simulink model "Final_EWASP_VC"  (R2022a)
settings: Solver=ode1  StartTime=0.0  StopTime=24*3600  FixedStep=10  RelTol=1e-3
values from neighbouring files (symbols this model uses):
  Aux_Threshold = 52    [Setup_Code_EWASP_VC.m]
  buildingAge = 2005    [Setup_Code_EWASP_VC.m]
  ceilingHeight = 2.4    [Setup_Code_EWASP_VC.m]
  conductiveHconnectMatrix = [ ... (first row only)    [Setup_Code_EWASP_VC.m]
  cRoofGreen = 100000    [Setup_Code_EWASP_VC.m]
  Defrost_After_Time = 30    [Setup_Code_EWASP_VC.m]
  DHWDemandProfile = occFreegainHotwaterElecTestPassiveOcc3(:,3)    [Setup_Code_EWASP_VC.m]
  Elec_Max = Elec_Max*(30/24.2)    [Setup_Code_EWASP_VC.m]
  Elec_Mid = Elec_Mid*(30/24.2)    [Setup_Code_EWASP_VC.m]
  Elec_Min = Elec_Min*(30/24.2)    [Setup_Code_EWASP_VC.m]
  ElecDemandProfile = occFreegainHotwaterElecTestPassiveOcc3(:,4)    [Setup_Code_EWASP_VC.m]
  ElecFixed = [Elec_Max(6,2) Elec_Max(6,4) Elec_Max(6,6) Elec_Max(6,7) ... (first row only)    [Setup_Code_EWASP_VC.m]
  floorOrCeilingArea = floorOrCeilingArea*1.15    [Setup_Code_EWASP_VC.m]
  forceCold = 0    [Setup_Code_EWASP_VC.m]
  freegain = occFreegainHotwaterElecTestPassiveOcc3(:,2)-max(occupancy)*25    [Setup_Code_EWASP_VC.m]
  furnitureModelOn = 1    [Setup_Code_EWASP_VC.m]
  Heat_Max = Heat_Max*(30/24.2)    [Setup_Code_EWASP_VC.m]
  Heat_Mid = Heat_Mid*(30/24.2)    [Setup_Code_EWASP_VC.m]
  Heat_Min = Heat_Min*(30/24.2)    [Setup_Code_EWASP_VC.m]
  HeatFixed = [Heat_Max(6,2) Heat_Max(6,4) Heat_Max(6,6) Heat_Max(6,7) ... (first row only)    [Setup_Code_EWASP_VC.m]
  HeatingOnProfile = repmat(HeatingOnProfile,365,1)    [Setup_Code_EWASP_VC.m]
  HEX_ReturnLowerLimit = 52.5    [Setup_Code_EWASP_VC.m]
  HEX_ReturnUpperLimit = 55    [Setup_Code_EWASP_VC.m]
  LeakMultiplier = 1+(2*(rand()-0.5)/10)    [Setup_Code_EWASP_VC.m]
  loopCap = 15    [Setup_Code_EWASP_VC.m]
  maxOcc = max(occupancyProfile)    [Setup_Code_EWASP_VC.m]
  NESW_wallArea = max(NESW_Lengths*ceilingHeight-NESW_Windows,0)    [Setup_Code_EWASP_VC.m]
  NESW_Windows = [ ... (first row only)    [Setup_Code_EWASP_VC.m]
  numRooms = roomCount    [Setup_Code_EWASP_VC.m]
  offsetDays = 0    [Setup_Code_EWASP_VC.m]
  pumpChoice = pumpChoices(MinIndex,1)    [Setup_Code_EWASP_VC.m]
  pumpRamp = 180    [Setup_Code_EWASP_VC.m]
  ReturnLowerLimit = 37.5    [Setup_Code_EWASP_VC.m]
  ReturnUpperLimit = 40    [Setup_Code_EWASP_VC.m]
  RoofIrradiance = Flat_NS_EW_RoofIrradiance(:,1)    [Setup_Code_EWASP_VC.m]
  roofStartTemp = ones(11,1)*20    [Setup_Code_EWASP_VC.m]
  rooftype = 0    [Setup_Code_EWASP_VC.m]
  RoomDataMatrix = [zeros(1,12);ones(1,12)*wallDensity;zeros(1,12);ones(1,12)*wallU;ones(1,12)*windowU;ones(1,12)*floorU;ones(1,12)*ceilingU;zeros(1,12);windowArea, 0;floorOrCeilingArea;zeros(1,12);floorOrCeilingArea*ceilingHeight]    [Setup_Code_EWASP_VC.m]
  roomVol = roomVol*1.15    [Setup_Code_EWASP_VC.m]
  slabStartTemp = (GroundTempTimeSeries(offsetDays*1440+1,1)+thermostatSetting)/2    [Setup_Code_EWASP_VC.m]
  SlackRequest = zeros(1440,1)    [Setup_Code_EWASP_VC.m]
  SolarThermalExists = 0    [Setup_Code_EWASP_VC.m]
  SourceFixed = HeatFixed-ElecFixed    [Setup_Code_EWASP_VC.m]
  StateSeries = StateSeriesGenerator(22,7,1)    [Setup_Code_EWASP_VC.m]
  Tank_Lower_Temp = 49.5    [Setup_Code_EWASP_VC.m]
  Tank_Upper_Temp = 52    [Setup_Code_EWASP_VC.m]
  Tank_Volume_m3 = 0.15    [Setup_Code_EWASP_VC.m]
  TankHeatHour = randi([1 5])-1    [Setup_Code_EWASP_VC.m]
  thermostatSetting = 20.0    (= 20)    [Setup_Code_EWASP_VC.m]
  upDown = [0;0;0;0;1;1;1;1;1;1;1]    [Setup_Code_EWASP_VC.m]
  variableASHP = 1    [Setup_Code_EWASP_VC.m]
  wallStartTempExt = thermostatSetting*(0.266+0.00215*outdoorStartTemp+0.018*wallU+0.00113*outdoorStartTemp*wallU+0.0068*wallU^2)    [Setup_Code_EWASP_VC.m]
undefined symbols (not defined in the file or in its folder): a, ceilingU, condUDMatrix, convUDMatrix, deltaPEXPANDED_E, deltaPEXPANDED_E2, deltaPEXPANDED_N, deltaPEXPANDED_N2, deltaPEXPANDED_S, deltaPEXPANDED_S2, deltaPEXPANDED_W, deltaPEXPANDED_W2, DesiredDHWTemp, DesiredFlowTempVsInOutDeltaTemp, DiffuseHorizontal, DiscIntNeverNeededParam, DNI, dwnAndConcrete, DWORK_A_HX, DWORK_CHK_FLU, DWORK_CP_NODE, DWORK_DH, DWORK_FLUID, DWORK_HCON, DWORK_LOSS, DWORK_MDOTDOWN, DWORK_MDOTIN, DWORK_MDOTUP, DWORK_MIX, DWORK_PRESS, DWORK_QDOTIN, DWORK_RHO_NODE, DWORK_TIN, DWORK_TS_OLD, DWORK_V_NODE, GroundTempTimeSeries, HCM, HCM2, HCM_closed, HCM_closed2, intermediateU, IsTop, massFlowMatrix, neighbourMatrix, numericalRoomUse, RadiatorMatrix, room2roomflowmatrix_E, room2roomflowmatrix_E2, room2roomflowmatrix_N, room2roomflowmatrix_N2, room2roomflowmatrix_S, room2roomflowmatrix_S2, room2roomflowmatrix_W, room2roomflowmatrix_W2, StateAirInEXPANDED_E, StateAirInEXPANDED_E2, StateAirInEXPANDED_N, StateAirInEXPANDED_N2, StateAirInEXPANDED_S, StateAirInEXPANDED_S2 ... (+23)
libraries: simulink x6, dspsigops x4, dspmtrx3 x4, carnot x3, spsEdgeDetectorLib x2, dspstat3 x2, powerlib_meascontrol x1, simulink_extras x1
(part 3 of 27)

== system Final_EWASP_VC/Subsystem_Room2 ==
  DNI2 : Constant  Value=0
  Diffuse Irradiance2 : Constant  Value=0
  Ground1 : Ground
  Incidence Angle2 : Constant  Value=60
  Integrator1 : Integrator  InitialConditionSource=external  InitialCondition=Tin1
  Kitchen : Subsystem
      mask Display:
      | port_label('input', 1, 'THB in')
      | port_label('input', 2, 'T In')
      | port_label('input', 3, 'T Out')
      | port_label('input', 4, 'T up (conv)')
      | port_label('input', 5, 'T Down (conv)')
      | port_label('input', 6, 'T Bel (cond)')
      | port_label('input', 7, 'T Abv (cond)')
      | port_label('input', 8, 'T N1')
      | port_label('input', 9, 'T N2')
      | port_label('input', 10, 'T N3')
      | port_label('input', 11, 'T N4')
      | port_label('input', 12, 'T N5')
      | port_label('input', 13, 'T Wall')
      | port_label('input', 14, 'Ang')
      | port_label('input', 15, 'Tilt')
      | port_label('input', 16, 'DNI')
      | port_label('input', 17, 'DiffI')
      | 
      | port_label('output', 1, 'THB Out')
      | 
      | port_label('output', 2, 'DeltaT Room')
      | 
      | port_label('input', 18, 'm_dot_Fully_open')
      | port_label('output', 3, 'm_dot_Actual')
  Panel TIlt2 : Constant  Value=90
  Subsystem10 : Subsystem
      mask Display:
      | disp('Vertical \n Conductive \n Signalling \n Block')
      | port_label('input', 1, 'Bel1')
      | port_label('input', 2, 'Bel2')
      | port_label('input', 3, 'Abv1')
      | port_label('input', 4, 'Abv2')
      | 
      | port_label('output', 1, 'T Bel')
      | port_label('output', 2, 'T Abv')
  Subsystem4 : Subsystem
      mask Display:
      | disp('Horizontal \n Neighbour \n Signalling \n Block')
      | port_label('input', 1, 'Nbr1')
      | port_label('input', 2, 'Nbr2')
      | port_label('input', 3, 'Nbr3')
      | port_label('input', 4, 'Nbr4')
      | port_label('input', 5, 'Nbr5')
      | port_label('output', 1, 'TN1')
      | port_label('output', 2, 'TN2')
      | port_label('output', 3, 'TN3')
      | port_label('output', 4, 'TN4')
      | port_label('output', 5, 'TN5')
  Terminator : Terminator
  Tinitial2 : Constant  Value=18
  Twall10 : Constant  Value=condUDMatrix(2,2)
  Twall128 : Constant  Value=neighbourMatrix(1,2)
  Twall129 : Constant  Value=neighbourMatrix(2,2)
  Twall130 : Constant  Value=neighbourMatrix(3,2)
  Twall131 : Constant  Value=neighbourMatrix(4,2)
  Twall132 : Constant  Value=neighbourMatrix(5,2)
  Twall31 : Constant  Value=condUDMatrix(3,3)
  Twall32 : Constant  Value=condUDMatrix(4,4)
  Twall9 : Constant  Value=condUDMatrix(1,2)
  tag scope: DeltaT_2=global, Mdot_Actual_2=global, T_2=global, T_return_R2=global
  wires:
  Subsystem10/2(Out2) -> Kitchen/7(In7)
  Twall9/1 -> Subsystem10/1(In1)
  Diffuse Irradiance2/1 -> Kitchen/17(In17)
  Twall10/1 -> Subsystem10/2(In2)
  Ground1/1 -> Kitchen/13(In13)
  [T_2] -> Kitchen/2(In2)
  [T_2] -> Kitchen/4(In4), Kitchen/5(In5)
  Subsystem4/3(Out3) -> Kitchen/10(In10)
  Subsystem10/1(Out1) -> Kitchen/6(In6)
  Twall32/1 -> Subsystem10/4(In4)
  [T_Out] -> Kitchen/3(In3)
  Incidence Angle2/1 -> Kitchen/14(In14)
  Twall31/1 -> Subsystem10/3(In3)
  Subsystem4/1(Out1) -> Kitchen/8(In8)
  Tinitial2/1 -> Integrator1/2
  Twall132/1 -> Subsystem4/5(In5)
  [DeltaT_2] -> Integrator1/1
  Twall130/1 -> Subsystem4/3(In3)
  Subsystem4/5(Out5) -> Kitchen/12(In12)
  Kitchen/2(Out3) -> [DeltaT_2]
  Kitchen/3(Out4) -> [Mdot_Actual_2]
  Kitchen/1(Out1) -> [T_return_R2]
  [MassFlow_Full_Open_2] -> Kitchen/18(In18)
  DNI2/1 -> Kitchen/16(In16)
  Subsystem4/2(Out2) -> Kitchen/9(In9)
  [THB_In] -> Kitchen/1(In1)
  Twall128/1 -> Subsystem4/1(In1)
  Twall131/1 -> Subsystem4/4(In4)
  Panel TIlt2/1 -> Kitchen/15(In15)
  Twall129/1 -> Subsystem4/2(In2)
  Integrator1/1 -> [T_2]
  Kitchen/4(Out2) -> Terminator/1
  Subsystem4/4(Out4) -> Kitchen/11(In11)

== system Final_EWASP_VC/Subsystem_Room3 ==
  DNI3 : Constant  Value=0
  Diffuse Irradiance3 : Constant  Value=50
  Ground2 : Ground
  Incidence Angle3 : Constant  Value=60
  Integrator5 : Integrator  InitialConditionSource=external  InitialCondition=Tin1
  Panel TIlt3 : Constant  Value=90
  Subsystem5 : Subsystem
      mask Display:
      | disp('Horizontal \n Neighbour \n Signalling \n Block')
      | port_label('input', 1, 'Nbr1')
      | port_label('input', 2, 'Nbr2')
      | port_label('input', 3, 'Nbr3')
      | port_label('input', 4, 'Nbr4')
      | port_label('input', 5, 'Nbr5')
      | port_label('output', 1, 'TN1')
      | port_label('output', 2, 'TN2')
      | port_label('output', 3, 'TN3')
      | port_label('output', 4, 'TN4')
      | port_label('output', 5, 'TN5')
  Subsystem9 : Subsystem
      mask Display:
      | disp('Vertical \n Conductive \n Signalling \n Block')
      | port_label('input', 1, 'Bel1')
      | port_label('input', 2, 'Bel2')
      | port_label('input', 3, 'Abv1')
      | port_label('input', 4, 'Abv2')
      | 
      | port_label('output', 1, 'T Bel')
      | port_label('output', 2, 'T Abv')
  Terminator11 : Terminator
  Tinitial3 : Constant  Value=18
  Twall16 : Constant  Value=neighbourMatrix(1,3)
  Twall17 : Constant  Value=neighbourMatrix(2,3)
  Twall18 : Constant  Value=neighbourMatrix(3,3)
  Twall19 : Constant  Value=neighbourMatrix(4,3)
  Twall20 : Constant  Value=neighbourMatrix(5,3)
  Twall5 : Constant  Value=condUDMatrix(1,3)
  Twall6 : Constant  Value=condUDMatrix(2,3)
  Twall7 : Constant  Value=condUDMatrix(3,3)
  Twall8 : Constant  Value=condUDMatrix(4,3)
  Utility : Subsystem
      mask Display:
      | port_label('input', 1, 'THB in')
      | port_label('input', 2, 'T In')
      | port_label('input', 3, 'T Out')
      | port_label('input', 4, 'T up (conv)')
      | port_label('input', 5, 'T Down (conv)')
      | port_label('input', 6, 'T Bel (cond)')
      | port_label('input', 7, 'T Abv (cond)')
      | port_label('input', 8, 'T N1')
      | port_label('input', 9, 'T N2')
      | port_label('input', 10, 'T N3')
      | port_label('input', 11, 'T N4')
      | port_label('input', 12, 'T N5')
      | port_label('input', 13, 'T Wall')
      | port_label('input', 14, 'Ang')
      | port_label('input', 15, 'Tilt')
      | port_label('input', 16, 'DNI')
      | port_label('input', 17, 'DiffI')
      | 
      | port_label('output', 1, 'THB Out')
      | port_label('output', 2, 'DeltaT Wall')
      | port_label('output', 3, 'DeltaT Room')
      | 
      | port_label('input', 18, 'm_dot_Fully_open')
      | port_label('output', 4, 'm_dot_Actual')
  tag scope: DeltaT_3=global, Mdot_Actual_3=global, T_3=global, T_return_R3=global
  wires:
  Ground2/1 -> Utility/13(In13)
  Subsystem5/3(Out3) -> Utility/10(In10)
  Twall5/1 -> Subsystem9/1(In1)
  Twall8/1 -> Subsystem9/4(In4)
  Twall6/1 -> Subsystem9/2(In2)
  Utility/2(Out2) -> Terminator11/1
  Twall7/1 -> Subsystem9/3(In3)
  [T_3] -> Utility/2(In2)
  Subsystem9/1(Out1) -> Utility/6(In6)
  Subsystem9/2(Out2) -> Utility/7(In7)
  Diffuse Irradiance3/1 -> Utility/17(In17)
  Integrator5/1 -> [T_3]
  Twall18/1 -> Subsystem5/3(In3)
  Incidence Angle3/1 -> Utility/14(In14)
  DNI3/1 -> Utility/16(In16)
  Panel TIlt3/1 -> Utility/15(In15)
  [THB_In] -> Utility/1(In1)
  Tinitial3/1 -> Integrator5/2
  Twall20/1 -> Subsystem5/5(In5)
  [T_Out] -> Utility/3(In3)
  [T_3] -> Utility/5(In5), Utility/4(In4)
  [MassFlow_Full_Open_3] -> Utility/18(In18)
  Utility/4(Out4) -> [Mdot_Actual_3]
  Utility/1(Out1) -> [T_return_R3]
  Twall16/1 -> Subsystem5/1(In1)
  Subsystem5/4(Out4) -> Utility/11(In11)
  Twall17/1 -> Subsystem5/2(In2)
  Subsystem5/2(Out2) -> Utility/9(In9)
  Utility/3(Out3) -> [DeltaT_3]
  Subsystem5/5(Out5) -> Utility/12(In12)
  [DeltaT_3] -> Integrator5/1
  Subsystem5/1(Out1) -> Utility/8(In8)
  Twall19/1 -> Subsystem5/4(In4)

== system Final_EWASP_VC/Subsystem_Room4 ==
  DNI11 : Constant  Value=0
  Diffuse Irradiance8 : Constant  Value=50
  Ground3 : Ground
  Hall : Subsystem
      mask Display:
      | port_label('input', 1, 'THB in')
      | port_label('input', 2, 'T In')
      | port_label('input', 3, 'T Out')
      | port_label('input', 4, 'T up (conv)')
      | port_label('input', 5, 'T Down (conv)')
      | port_label('input', 6, 'T Bel (cond)')
      | port_label('input', 7, 'T Abv (cond)')
      | port_label('input', 8, 'T N1')
      | port_label('input', 9, 'T N2')
      | port_label('input', 10, 'T N3')
      | port_label('input', 11, 'T N4')
      | port_label('input', 12, 'T N5')
      | port_label('input', 13, 'T Wall')
      | port_label('input', 14, 'Ang')
      | port_label('input', 15, 'Tilt')
      | port_label('input', 16, 'DNI')
      | port_label('input', 17, 'DiffI')
      | 
      | port_label('output', 1, 'THB Out')
      | port_label('output', 2, 'DeltaT Wall')
      | port_label('output', 3, 'DeltaT Room')
      | 
      | 
      | port_label('input', 18, 'm_dot_Fully_open')
      | port_label('output', 4, 'm_dot_Actual')
  Incidence Angle8 : Constant  Value=60
  Integrator21 : Integrator  InitialConditionSource=external  InitialCondition=Tin1
  Panel TIlt8 : Constant  Value=90
  Subsystem6 : Subsystem
      mask Display:
      | disp('Horizontal \n Neighbour \n Signalling \n Block')
      | port_label('input', 1, 'Nbr1')
      | port_label('input', 2, 'Nbr2')
      | port_label('input', 3, 'Nbr3')
      | port_label('input', 4, 'Nbr4')
      | port_label('input', 5, 'Nbr5')
      | port_label('output', 1, 'TN1')
      | port_label('output', 2, 'TN2')
      | port_label('output', 3, 'TN3')
      | port_label('output', 4, 'TN4')
      | port_label('output', 5, 'TN5')
  Subsystem8 : Subsystem
      mask Display:
      | disp('Vertical \n Conductive \n Signalling \n Block')
      | port_label('input', 1, 'Bel1')
      | port_label('input', 2, 'Bel2')
      | port_label('input', 3, 'Abv1')
      | port_label('input', 4, 'Abv2')
      | 
      | port_label('output', 1, 'T Bel')
      | port_label('output', 2, 'T Abv')
  Terminator10 : Terminator
  Tinitial11 : Constant  Value=18
  Twall1 : Constant  Value=condUDMatrix(1,4)
  Twall2 : Constant  Value=condUDMatrix(2,4)
  Twall21 : Constant  Value=neighbourMatrix(1,4)
  Twall22 : Constant  Value=neighbourMatrix(2,4)
  Twall23 : Constant  Value=neighbourMatrix(3,4)
  Twall24 : Constant  Value=neighbourMatrix(4,4)
  Twall25 : Constant  Value=neighbourMatrix(5,4)
  Twall3 : Constant  Value=condUDMatrix(3,4)
  Twall4 : Constant  Value=condUDMatrix(4,4)
  tag scope: DeltaT_4=global, Mdot_Actual_4=global, T_4=global, T_return_R4=global
  wires:
  Subsystem8/2(Out2) -> Hall/7(In7)
  Integrator21/1 -> [T_4]
  Subsystem6/1(Out1) -> Hall/8(In8)
  Ground3/1 -> Hall/13(In13)
  [DeltaT_4] -> Integrator21/1
  Incidence Angle8/1 -> Hall/14(In14)
  Subsystem8/1(Out1) -> Hall/6(In6)
  Panel TIlt8/1 -> Hall/15(In15)
  [THB_In] -> Hall/1(In1)
  Twall21/1 -> Subsystem6/1(In1)
  DNI11/1 -> Hall/16(In16)
  Diffuse Irradiance8/1 -> Hall/17(In17)
  Hall/4(Out4) -> [Mdot_Actual_4]
  Hall/3(Out3) -> [DeltaT_4]
  Twall25/1 -> Subsystem6/5(In5)
  [MassFlow_Full_Open_4] -> Hall/18(In18)
  Twall23/1 -> Subsystem6/3(In3)
  Subsystem6/5(Out5) -> Hall/12(In12)
  Twall4/1 -> Subsystem8/4(In4)
  Twall2/1 -> Subsystem8/2(In2)
  [T_4] -> Hall/5(In5)
  Hall/2(Out2) -> Terminator10/1
  [T_4] -> Hall/2(In2)
  Subsystem6/4(Out4) -> Hall/11(In11)
  Subsystem6/3(Out3) -> Hall/10(In10)
  Twall24/1 -> Subsystem6/4(In4)
  Twall22/1 -> Subsystem6/2(In2)
  Hall/1(Out1) -> [T_return_R4]
  Subsystem6/2(Out2) -> Hall/9(In9)
  Tinitial11/1 -> Integrator21/2
  [T_5] -> Hall/4(In4)
  Twall1/1 -> Subsystem8/1(In1)
  [T_Out] -> Hall/3(In3)
  Twall3/1 -> Subsystem8/3(In3)

== system Final_EWASP_VC/Subsystem_Room5 ==
  DNI4 : Constant  Value=0
  Diffuse Irradiance4 : Constant  Value=0
  Ground4 : Ground
  Incidence Angle4 : Constant  Value=60
  Integrator6 : Integrator  InitialConditionSource=external  InitialCondition=Tin1
  Landing : Subsystem
      mask Display:
      | port_label('input', 1, 'THB in')
      | port_label('input', 2, 'T In')
      | port_label('input', 3, 'T Out')
      | port_label('input', 4, 'T up (conv)')
      | port_label('input', 5, 'T Down (conv)')
      | port_label('input', 6, 'T Bel (cond)')
      | port_label('input', 7, 'T Abv (cond)')
      | port_label('input', 8, 'T N1')
      | port_label('input', 9, 'T N2')
      | port_label('input', 10, 'T N3')
      | port_label('input', 11, 'T N4')
      | port_label('input', 12, 'T N5')
      | port_label('input', 13, 'T Wall')
      | port_label('input', 14, 'Ang')
      | port_label('input', 15, 'Tilt')
      | port_label('input', 16, 'DNI')
      | port_label('input', 17, 'DiffI')
      | 
      | port_label('output', 1, 'THB Out')
      | port_label('output', 2, 'DeltaT Wall')
      | port_label('output', 3, 'DeltaT Room')
      | 
      | port_label('input', 18, 'm_dot_Fully_open')
      | port_label('output', 5, 'm_dot_Actual')
  Panel TIlt4 : Constant  Value=90
  Subsystem18 : Subsystem
      mask Display:
      | disp('Vertical \n Convective \n Signalling \n Block')
      | port_label('input', 1, 'Nbr1')
      | port_label('input', 2, 'Nbr2')
      | 
      | port_label('output', 1, 'Tup')
      | port_label('output', 2, 'Tdwn')
  Subsystem35 : Subsystem
      mask Display:
      | disp('Vertical \n Conductive \n Signalling \n Block')
      | port_label('input', 1, 'Bel1')
      | port_label('input', 2, 'Bel2')
      | port_label('input', 3, 'Abv1')
      | port_label('input', 4, 'Abv2')
      | 
      | port_label('output', 1, 'T Bel')
      | port_label('output', 2, 'T Abv')
  Subsystem7 : Subsystem
      mask Display:
      | disp('Horizontal \n Neighbour \n Signalling \n Block')
      | port_label('input', 1, 'Nbr1')
      | port_label('input', 2, 'Nbr2')
      | port_label('input', 3, 'Nbr3')
      | port_label('input', 4, 'Nbr4')
      | port_label('input', 5, 'Nbr5')
      | port_label('output', 1, 'TN1')
      | port_label('output', 2, 'TN2')
      | port_label('output', 3, 'TN3')
      | port_label('output', 4, 'TN4')
      | port_label('output', 5, 'TN5')
  Terminator12 : Terminator
  Terminator9 : Terminator
  Tinitial4 : Constant  Value=18
  Twall104 : Constant  Value=convUDMatrix(1,5)
  Twall105 : Constant  Value=convUDMatrix(2,5)
  Twall119 : Constant  Value=condUDMatrix(1,5)
  Twall120 : Constant  Value=condUDMatrix(2,5)
  Twall121 : Constant  Value=condUDMatrix(3,5)
  Twall122 : Constant  Value=condUDMatrix(4,5)
  Twall26 : Constant  Value=neighbourMatrix(1,5)
  Twall27 : Constant  Value=neighbourMatrix(2,5)
  Twall28 : Constant  Value=neighbourMatrix(3,5)
  Twall29 : Constant  Value=neighbourMatrix(4,5)
  Twall30 : Constant  Value=neighbourMatrix(5,5)
  tag scope: DeltaT_5=global, Mdot_Actual_5=global, T_5=global, T_return_R5=global
  wires:
  DNI4/1 -> Landing/16(In16)
  Twall120/1 -> Subsystem35/2(In2)
  Tinitial4/1 -> Integrator6/2
  [DeltaT_5] -> Integrator6/1
  Landing/3(Out3) -> [DeltaT_5]
  Subsystem7/5(Out5) -> Landing/12(In12)
  Integrator6/1 -> [T_5]
  Subsystem7/1(Out1) -> Landing/8(In8)
  Twall119/1 -> Subsystem35/1(In1)
  Diffuse Irradiance4/1 -> Landing/17(In17)
  Panel TIlt4/1 -> Landing/15(In15)
  [THB_In] -> Landing/1(In1)
  [T_Out] -> Landing/3(In3)
  Landing/5(Out5) -> [Mdot_Actual_5]
  Incidence Angle4/1 -> Landing/14(In14)
  Subsystem35/1(Out1) -> Landing/6(In6)
  Twall26/1 -> Subsystem7/1(In1)
  [T_5] -> Landing/2(In2)
  Ground4/1 -> Landing/13(In13)
  Subsystem7/3(Out3) -> Landing/10(In10)
  [MassFlow_Full_Open_5] -> Landing/18(In18)
  Twall27/1 -> Subsystem7/2(In2)
  Twall121/1 -> Subsystem35/3(In3)
  Subsystem18/2(Out2) -> Landing/5(In5)
  Subsystem18/1(Out1) -> Landing/4(In4)
  Twall122/1 -> Subsystem35/4(In4)
  Landing/4(Out4) -> Terminator12/1
  Landing/2(Out2) -> Terminator9/1
  Twall105/1 -> Subsystem18/2(In2)
  Subsystem7/4(Out4) -> Landing/11(In11)
  Subsystem35/2(Out2) -> Landing/7(In7)
  Landing/1(Out1) -> [T_return_R5]
  Twall30/1 -> Subsystem7/5(In5)
  Twall28/1 -> Subsystem7/3(In3)
  Twall104/1 -> Subsystem18/1(In1)
  Twall29/1 -> Subsystem7/4(In4)
  Subsystem7/2(Out2) -> Landing/9(In9)

== system Final_EWASP_VC/Subsystem_Room6 ==
  Bedroom1 : Subsystem
      mask Display:
      | port_label('input', 1, 'THB in')
      | port_label('input', 2, 'T In')
      | port_label('input', 3, 'T Out')
      | port_label('input', 4, 'T up (conv)')
      | port_label('input', 5, 'T Down (conv)')
      | port_label('input', 6, 'T Bel (cond)')
      | port_label('input', 7, 'T Abv (cond)')
      | port_label('input', 8, 'T N1')
      | port_label('input', 9, 'T N2')
      | port_label('input', 10, 'T N3')
      | port_label('input', 11, 'T N4')
      | port_label('input', 12, 'T N5')
      | port_label('input', 13, 'T Wall')
      | port_label('input', 14, 'Ang')
      | port_label('input', 15, 'Tilt')
      | port_label('input', 16, 'DNI')
      | port_label('input', 17, 'DiffI')
      | 
      | port_label('output', 1, 'THB Out')
      | port_label('output', 2, 'DeltaT Wall')
      | port_label('output', 3, 'DeltaT Room')
      | 
      | port_label('input', 18, 'm_dot_Fully_open')
      | port_label('output', 5, 'm_dot_Actual')
  DNI5 : Constant  Value=0
  Diffuse Irradiance5 : Constant  Value=0
  Ground10 : Ground
  Incidence Angle5 : Constant  Value=60
  Integrator7 : Integrator  InitialConditionSource=external  InitialCondition=Tin1
  Panel TIlt5 : Constant  Value=90
  Scope38 : Scope
  Subsystem19 : Subsystem
      mask Display:
      | disp('Vertical \n Convective \n Signalling \n Block')
      | port_label('input', 1, 'Nbr1')
      | port_label('input', 2, 'Nbr2')
      | 
      | port_label('output', 1, 'Tup')
      | port_label('output', 2, 'Tdwn')
  Subsystem30 : Subsystem
      mask Display:
      | disp('Vertical \n Conductive \n Signalling \n Block')
      | port_label('input', 1, 'Bel1')
      | port_label('input', 2, 'Bel2')
      | port_label('input', 3, 'Abv1')
      | port_label('input', 4, 'Abv2')
      | 
      | port_label('output', 1, 'T Bel')
      | port_label('output', 2, 'T Abv')
  Subsystem8 : Subsystem
      mask Display:
      | disp('Horizontal \n Neighbour \n Signalling \n Block')
      | port_label('input', 1, 'Nbr1')
      | port_label('input', 2, 'Nbr2')
      | port_label('input', 3, 'Nbr3')
      | port_label('input', 4, 'Nbr4')
      | port_label('input', 5, 'Nbr5')
      | port_label('output', 1, 'TN1')
      | port_label('output', 2, 'TN2')
      | port_label('output', 3, 'TN3')
      | port_label('output', 4, 'TN4')
      | port_label('output', 5, 'TN5')
  Terminator4 : Terminator
  Tinitial5 : Constant  Value=18
  Twall108 : Constant  Value=condUDMatrix(1,6)
  Twall109 : Constant  Value=condUDMatrix(2,6)
  Twall110 : Constant  Value=condUDMatrix(3,6)
  Twall111 : Constant  Value=condUDMatrix(4,6)
  Twall31 : Constant  Value=neighbourMatrix(1,6)
  Twall32 : Constant  Value=neighbourMatrix(2,6)
  Twall33 : Constant  Value=neighbourMatrix(3,6)
  Twall34 : Constant  Value=neighbourMatrix(4,6)
  Twall35 : Constant  Value=neighbourMatrix(5,6)
  Twall74 : Constant  Value=convUDMatrix(1,6)
  Twall75 : Constant  Value=convUDMatrix(2,6)
  tag scope: DeltaT_6=global, Mdot_Actual_6=global, T_6=global, T_return_R6=global
  wires:
  Twall75/1 -> Subsystem19/2(In2)
  Subsystem8/1(Out1) -> Bedroom1/8(In8)
  DNI5/1 -> Bedroom1/16(In16)
  Subsystem19/2(Out2) -> Bedroom1/5(In5)
  [THB_In] -> Bedroom1/1(In1)
  Integrator7/1 -> [T_6]
  [T_6] -> Bedroom1/2(In2)
  Twall31/1 -> Subsystem8/1(In1)
  [DeltaT_6] -> Integrator7/1
  Subsystem19/1(Out1) -> Bedroom1/4(In4)
  Twall34/1 -> Subsystem8/4(In4)
  Incidence Angle5/1 -> Bedroom1/14(In14)
  Twall108/1 -> Subsystem30/1(In1)
  Ground10/1 -> Bedroom1/13(In13)
  [T_Out] -> Bedroom1/3(In3)
  Panel TIlt5/1 -> Bedroom1/15(In15)
  Bedroom1/3(Out3) -> [DeltaT_6]
  Bedroom1/4(Out4) -> Scope38/1
  Tinitial5/1 -> Integrator7/2
  Bedroom1/5(Out5) -> [Mdot_Actual_6]
  Bedroom1/1(Out1) -> [T_return_R6]
  [MassFlow_Full_Open_6] -> Bedroom1/18(In18)
  Twall110/1 -> Subsystem30/3(In3)
  Subsystem8/3(Out3) -> Bedroom1/10(In10)
  Subsystem8/2(Out2) -> Bedroom1/9(In9)
  Subsystem8/5(Out5) -> Bedroom1/12(In12)
  Twall35/1 -> Subsystem8/5(In5)
  Twall32/1 -> Subsystem8/2(In2)
  Twall111/1 -> Subsystem30/4(In4)
  Twall74/1 -> Subsystem19/1(In1)
  Diffuse Irradiance5/1 -> Bedroom1/17(In17)
  Twall33/1 -> Subsystem8/3(In3)
  Subsystem8/4(Out4) -> Bedroom1/11(In11)
  Subsystem30/1(Out1) -> Bedroom1/6(In6)
  Bedroom1/2(Out2) -> Terminator4/1
  Twall109/1 -> Subsystem30/2(In2)
  Subsystem30/2(Out2) -> Bedroom1/7(In7)

== system Final_EWASP_VC/Subsystem_Room7 ==
  Bedroom 2 : Subsystem
      mask Display:
      | port_label('input', 1, 'THB in')
      | port_label('input', 2, 'T In')
      | port_label('input', 3, 'T Out')
      | port_label('input', 4, 'T up (conv)')
      | port_label('input', 5, 'T Down (conv)')
      | port_label('input', 6, 'T Bel (cond)')
      | port_label('input', 7, 'T Abv (cond)')
      | port_label('input', 8, 'T N1')
      | port_label('input', 9, 'T N2')
      | port_label('input', 10, 'T N3')
      | port_label('input', 11, 'T N4')
      | port_label('input', 12, 'T N5')
      | port_label('input', 13, 'T Wall')
      | port_label('input', 14, 'Ang')
      | port_label('input', 15, 'Tilt')
      | port_label('input', 16, 'DNI')
      | port_label('input', 17, 'DiffI')
      | 
      | port_label('output', 1, 'THB Out')
      | port_label('output', 2, 'DeltaT Wall')
      | port_label('output', 3, 'DeltaT Room')
      | 
      | port_label('input', 18, 'm_dot_Fully_open')
      | port_label('output', 5, 'm_dot_Actual')
  DNI6 : Constant  Value=0
  Diffuse Irradiance6 : Constant  Value=0
  Ground9 : Ground
  Incidence Angle6 : Constant  Value=60
  Integrator11 : Integrator  InitialConditionSource=external  InitialCondition=Tin1
  Panel TIlt6 : Constant  Value=90
  Scope37 : Scope
  Subsystem20 : Subsystem
      mask Display:
      | disp('Vertical \n Convective \n Signalling \n Block')
      | port_label('input', 1, 'Nbr1')
      | port_label('input', 2, 'Nbr2')
      | 
      | port_label('output', 1, 'Tup')
      | port_label('output', 2, 'Tdwn')
  Subsystem25 : Subsystem
      mask Display:
      | disp('Vertical \n Conductive \n Signalling \n Block')
      | port_label('input', 1, 'Bel1')
      | port_label('input', 2, 'Bel2')
      | port_label('input', 3, 'Abv1')
      | port_label('input', 4, 'Abv2')
      | 
      | port_label('output', 1, 'T Bel')
      | port_label('output', 2, 'T Abv')
  Subsystem9 : Subsystem
      mask Display:
      | disp('Horizontal \n Neighbour \n Signalling \n Block')
      | port_label('input', 1, 'Nbr1')
      | port_label('input', 2, 'Nbr2')
      | port_label('input', 3, 'Nbr3')
      | port_label('input', 4, 'Nbr4')
      | port_label('input', 5, 'Nbr5')
      | port_label('output', 1, 'TN1')
      | port_label('output', 2, 'TN2')
      | port_label('output', 3, 'TN3')
      | port_label('output', 4, 'TN4')
      | port_label('output', 5, 'TN5')
  Terminator3 : Terminator
  Tinitial6 : Constant  Value=18
  Twall36 : Constant  Value=neighbourMatrix(1,7)
  Twall37 : Constant  Value=neighbourMatrix(2,7)
  Twall38 : Constant  Value=neighbourMatrix(3,7)
  Twall39 : Constant  Value=neighbourMatrix(4,7)
  Twall40 : Constant  Value=neighbourMatrix(5,7)
  Twall76 : Constant  Value=convUDMatrix(1,7)
  Twall77 : Constant  Value=convUDMatrix(2,7)
  Twall88 : Constant  Value=condUDMatrix(1,7)
  Twall89 : Constant  Value=condUDMatrix(2,7)
  Twall90 : Constant  Value=condUDMatrix(3,7)
  Twall91 : Constant  Value=condUDMatrix(4,7)
  tag scope: DeltaT_7=global, Mdot_Actual_7=global, T_7=global, T_return_R7=global
  wires:
  Panel TIlt6/1 -> Bedroom 2/15(In15)
  [T_Out] -> Bedroom 2/3(In3)
  Twall36/1 -> Subsystem9/1(In1)
  Bedroom 2/3(Out3) -> [DeltaT_7]
  [MassFlow_Full_Open_7] -> Bedroom 2/18(In18)
  Diffuse Irradiance6/1 -> Bedroom 2/17(In17)
  Bedroom 2/1(Out1) -> [T_return_R7]
  Bedroom 2/2(Out2) -> Terminator3/1
  Twall88/1 -> Subsystem25/1(In1)
  Subsystem9/3(Out3) -> Bedroom 2/10(In10)
  Bedroom 2/5(Out5) -> [Mdot_Actual_7]
  Twall90/1 -> Subsystem25/3(In3)
  Subsystem25/2(Out2) -> Bedroom 2/7(In7)
  Incidence Angle6/1 -> Bedroom 2/14(In14)
  DNI6/1 -> Bedroom 2/16(In16)
  Integrator11/1 -> [T_7]
  Subsystem9/1(Out1) -> Bedroom 2/8(In8)
  Subsystem25/1(Out1) -> Bedroom 2/6(In6)
  [DeltaT_7] -> Integrator11/1
  Twall40/1 -> Subsystem9/5(In5)
  Subsystem20/1(Out1) -> Bedroom 2/4(In4)
  Tinitial6/1 -> Integrator11/2
  Twall37/1 -> Subsystem9/2(In2)
  Subsystem20/2(Out2) -> Bedroom 2/5(In5)
  Bedroom 2/4(Out4) -> Scope37/1
  [THB_In] -> Bedroom 2/1(In1)
  Twall76/1 -> Subsystem20/1(In1)
  Subsystem9/4(Out4) -> Bedroom 2/11(In11)
  [T_7] -> Bedroom 2/2(In2)
  Subsystem9/2(Out2) -> Bedroom 2/9(In9)
  Twall39/1 -> Subsystem9/4(In4)
  Twall89/1 -> Subsystem25/2(In2)
  Ground9/1 -> Bedroom 2/13(In13)
  Twall38/1 -> Subsystem9/3(In3)
  Subsystem9/5(Out5) -> Bedroom 2/12(In12)
  Twall91/1 -> Subsystem25/4(In4)
  Twall77/1 -> Subsystem20/2(In2)

== system Final_EWASP_VC/Subsystem_Room8 ==
  Bedroom3 : Subsystem
      mask Display:
      | port_label('input', 1, 'THB in')
      | port_label('input', 2, 'T In')
      | port_label('input', 3, 'T Out')
      | port_label('input', 4, 'T up (conv)')
      | port_label('input', 5, 'T Down (conv)')
      | port_label('input', 6, 'T Bel (cond)')
      | port_label('input', 7, 'T Abv (cond)')
      | port_label('input', 8, 'T N1')
      | port_label('input', 9, 'T N2')
      | port_label('input', 10, 'T N3')
      | port_label('input', 11, 'T N4')
      | port_label('input', 12, 'T N5')
      | port_label('input', 13, 'T Wall')
      | port_label('input', 14, 'Ang')
      | port_label('input', 15, 'Tilt')
      | port_label('input', 16, 'DNI')
      | port_label('input', 17, 'DiffI')
      | 
      | port_label('output', 1, 'THB Out')
      | port_label('output', 2, 'DeltaT Wall')
      | port_label('output', 3, 'DeltaT Room')
      | 
      | port_label('input', 18, 'm_dot_Fully_open')
      | port_label('output', 5, 'm_dot_Actual')
  DNI7 : Constant  Value=0
  Diffuse Irradiance7 : Constant  Value=0
  Ground8 : Ground
  Incidence Angle7 : Constant  Value=60
  Integrator13 : Integrator  InitialConditionSource=external  InitialCondition=Tin1
  Panel TIlt7 : Constant  Value=90
  Scope36 : Scope
  Subsystem10 : Subsystem
      mask Display:
      | disp('Horizontal \n Neighbour \n Signalling \n Block')
      | port_label('input', 1, 'Nbr1')
      | port_label('input', 2, 'Nbr2')
      | port_label('input', 3, 'Nbr3')
      | port_label('input', 4, 'Nbr4')
      | port_label('input', 5, 'Nbr5')
      | port_label('output', 1, 'TN1')
      | port_label('output', 2, 'TN2')
      | port_label('output', 3, 'TN3')
      | port_label('output', 4, 'TN4')
      | port_label('output', 5, 'TN5')
  Subsystem21 : Subsystem
      mask Display:
      | disp('Vertical \n Convective \n Signalling \n Block')
      | port_label('input', 1, 'Nbr1')
      | port_label('input', 2, 'Nbr2')
      | 
      | port_label('output', 1, 'Tup')
      | port_label('output', 2, 'Tdwn')
  Subsystem26 : Subsystem
      mask Display:
      | disp('Vertical \n Conductive \n Signalling \n Block')
      | port_label('input', 1, 'Bel1')
      | port_label('input', 2, 'Bel2')
      | port_label('input', 3, 'Abv1')
      | port_label('input', 4, 'Abv2')
      | 
      | port_label('output', 1, 'T Bel')
      | port_label('output', 2, 'T Abv')
  Terminator5 : Terminator
  Tinitial7 : Constant  Value=18
  Twall41 : Constant  Value=neighbourMatrix(1,8)
  Twall42 : Constant  Value=neighbourMatrix(2,8)
  Twall43 : Constant  Value=neighbourMatrix(3,8)
  Twall44 : Constant  Value=neighbourMatrix(4,8)
  Twall45 : Constant  Value=neighbourMatrix(5,8)
  Twall78 : Constant  Value=convUDMatrix(1,8)
  Twall79 : Constant  Value=convUDMatrix(2,8)
  Twall92 : Constant  Value=condUDMatrix(1,8)
  Twall93 : Constant  Value=condUDMatrix(2,8)
  Twall94 : Constant  Value=condUDMatrix(3,8)
  Twall95 : Constant  Value=condUDMatrix(4,8)
  tag scope: DeltaT_8=global, Mdot_Actual_8=global, T_8=global, T_return_R8=global
  wires:
  [THB_In] -> Bedroom3/1(In1)
  [T_8] -> Bedroom3/2(In2)
  Integrator13/1 -> [T_8]
  Ground8/1 -> Bedroom3/13(In13)
  Subsystem10/5(Out5) -> Bedroom3/12(In12)
  Tinitial7/1 -> Integrator13/2
  Subsystem26/1(Out1) -> Bedroom3/6(In6)
  Twall41/1 -> Subsystem10/1(In1)
  [T_Out] -> Bedroom3/3(In3)
  Subsystem10/3(Out3) -> Bedroom3/10(In10)
  Diffuse Irradiance7/1 -> Bedroom3/17(In17)
  Subsystem10/2(Out2) -> Bedroom3/9(In9)
  Subsystem21/1(Out1) -> Bedroom3/4(In4)
  DNI7/1 -> Bedroom3/16(In16)
  Twall94/1 -> Subsystem26/3(In3)
  Bedroom3/2(Out2) -> Terminator5/1
  [MassFlow_Full_Open_8] -> Bedroom3/18(In18)
  Bedroom3/5(Out5) -> [Mdot_Actual_8]
  Incidence Angle7/1 -> Bedroom3/14(In14)
  Bedroom3/3(Out3) -> [DeltaT_8]
  Subsystem10/4(Out4) -> Bedroom3/11(In11)
  Panel TIlt7/1 -> Bedroom3/15(In15)
  Twall45/1 -> Subsystem10/5(In5)
  Twall79/1 -> Subsystem21/2(In2)
  Twall93/1 -> Subsystem26/2(In2)
  Subsystem21/2(Out2) -> Bedroom3/5(In5)
  Twall92/1 -> Subsystem26/1(In1)
  Twall43/1 -> Subsystem10/3(In3)
  Twall44/1 -> Subsystem10/4(In4)
  Twall42/1 -> Subsystem10/2(In2)
  Subsystem10/1(Out1) -> Bedroom3/8(In8)
  Bedroom3/1(Out1) -> [T_return_R8]
  Subsystem26/2(Out2) -> Bedroom3/7(In7)
  [DeltaT_8] -> Integrator13/1
  Twall95/1 -> Subsystem26/4(In4)
  Twall78/1 -> Subsystem21/1(In1)
  Bedroom3/4(Out4) -> Scope36/1

== system Final_EWASP_VC/Subsystem_Room9 ==
  Bedroom4 : Subsystem
      mask Display:
      | port_label('input', 1, 'THB in')
      | port_label('input', 2, 'T In')
      | port_label('input', 3, 'T Out')
      | port_label('input', 4, 'T up (conv)')
      | port_label('input', 5, 'T Down (conv)')
      | port_label('input', 6, 'T Bel (cond)')
      | port_label('input', 7, 'T Abv (cond)')
      | port_label('input', 8, 'T N1')
      | port_label('input', 9, 'T N2')
      | port_label('input', 10, 'T N3')
      | port_label('input', 11, 'T N4')
      | port_label('input', 12, 'T N5')
      | port_label('input', 13, 'T Wall')
      | port_label('input', 14, 'Ang')
      | port_label('input', 15, 'Tilt')
      | port_label('input', 16, 'DNI')
      | port_label('input', 17, 'DiffI')
      | 
      | port_label('output', 1, 'THB Out')
      | port_label('output', 2, 'DeltaT Wall')
      | port_label('output', 3, 'DeltaT Room')
      | 
      | port_label('input', 18, 'm_dot_Fully_open')
      | port_label('output', 5, 'm_dot_Actual')
  DNI13 : Constant  Value=0
  Diffuse Irradiance9 : Constant  Value=0
  Ground7 : Ground
  Incidence Angle9 : Constant  Value=60
  Integrator18 : Integrator  InitialConditionSource=external  InitialCondition=Tin1
  Panel TIlt9 : Constant  Value=90
  Scope35 : Scope
  Subsystem11 : Subsystem
      mask Display:
      | disp('Horizontal \n Neighbour \n Signalling \n Block')
      | port_label('input', 1, 'Nbr1')
      | port_label('input', 2, 'Nbr2')
      | port_label('input', 3, 'Nbr3')
      | port_label('input', 4, 'Nbr4')
      | port_label('input', 5, 'Nbr5')
      | port_label('output', 1, 'TN1')
      | port_label('output', 2, 'TN2')
      | port_label('output', 3, 'TN3')
      | port_label('output', 4, 'TN4')
      | port_label('output', 5, 'TN5')
  Subsystem22 : Subsystem
      mask Display:
      | disp('Vertical \n Convective \n Signalling \n Block')
      | port_label('input', 1, 'Nbr1')
      | port_label('input', 2, 'Nbr2')
      | 
      | port_label('output', 1, 'Tup')
      | port_label('output', 2, 'Tdwn')
  Subsystem27 : Subsystem
      mask Display:
      | disp('Vertical \n Conductive \n Signalling \n Block')
      | port_label('input', 1, 'Bel1')
      | port_label('input', 2, 'Bel2')
      | port_label('input', 3, 'Abv1')
      | port_label('input', 4, 'Abv2')
      | 
      | port_label('output', 1, 'T Bel')
      | port_label('output', 2, 'T Abv')
  Terminator6 : Terminator
  Tinitial13 : Constant  Value=18
  Twall46 : Constant  Value=neighbourMatrix(1,9)
  Twall47 : Constant  Value=neighbourMatrix(2,9)
  Twall48 : Constant  Value=neighbourMatrix(3,9)
  Twall49 : Constant  Value=neighbourMatrix(4,9)
  Twall50 : Constant  Value=neighbourMatrix(5,9)
  Twall80 : Constant  Value=convUDMatrix(1,9)
  Twall81 : Constant  Value=convUDMatrix(2,9)
  Twall96 : Constant  Value=condUDMatrix(1,9)
  Twall97 : Constant  Value=condUDMatrix(2,9)
  Twall98 : Constant  Value=condUDMatrix(3,9)
  Twall99 : Constant  Value=condUDMatrix(4,9)
  tag scope: DeltaT_9=global, Mdot_Actual_9=global, T_9=global, T_return_R9=global
  wires:
  Twall47/1 -> Subsystem11/2(In2)
  [DeltaT_9] -> Integrator18/1
  [THB_In] -> Bedroom4/1(In1)
  Twall46/1 -> Subsystem11/1(In1)
  Subsystem22/2(Out2) -> Bedroom4/5(In5)
  Integrator18/1 -> [T_9]
  Tinitial13/1 -> Integrator18/2
  Diffuse Irradiance9/1 -> Bedroom4/17(In17)
  Incidence Angle9/1 -> Bedroom4/14(In14)
  Bedroom4/3(Out3) -> [DeltaT_9]
  Subsystem11/2(Out2) -> Bedroom4/9(In9)
  Bedroom4/1(Out1) -> [T_return_R9]
  Twall80/1 -> Subsystem22/1(In1)
  Bedroom4/4(Out4) -> Scope35/1
  Bedroom4/2(Out2) -> Terminator6/1
  Subsystem22/1(Out1) -> Bedroom4/4(In4)
  Subsystem11/1(Out1) -> Bedroom4/8(In8)
  Subsystem27/2(Out2) -> Bedroom4/7(In7)
  Subsystem11/3(Out3) -> Bedroom4/10(In10)
  Twall48/1 -> Subsystem11/3(In3)
  [T_9] -> Bedroom4/2(In2)
  Twall96/1 -> Subsystem27/1(In1)
  Twall49/1 -> Subsystem11/4(In4)
  Subsystem11/5(Out5) -> Bedroom4/12(In12)
  Twall98/1 -> Subsystem27/3(In3)
  Subsystem27/1(Out1) -> Bedroom4/6(In6)
  [T_Out] -> Bedroom4/3(In3)
  Twall99/1 -> Subsystem27/4(In4)
  Twall81/1 -> Subsystem22/2(In2)
  Panel TIlt9/1 -> Bedroom4/15(In15)
  Twall97/1 -> Subsystem27/2(In2)
  Twall50/1 -> Subsystem11/5(In5)
  Ground7/1 -> Bedroom4/13(In13)
  [MassFlow_Full_Open_9] -> Bedroom4/18(In18)
  DNI13/1 -> Bedroom4/16(In16)
  Subsystem11/4(Out4) -> Bedroom4/11(In11)
  Bedroom4/5(Out5) -> [Mdot_Actual_9]
